simulink model "audio_project"  (R2022b)
settings: Solver=FixedStepDiscrete  StartTime=0.0  StopTime=inf  RelTol=1e-3
model workspace (MAT data in the model file):
  L = 5
  R = 0.5
  p = 2
libraries: audiosources x2, dspsnks4 x1
settings Model: Creator=The MathWorks, Inc.  LastModifiedBy=aymer
settings SolverCC: AlgebraicLoopSolver=TrustRegion  AutoInsertRateTranBlk=on
settings DataIOCC: LimitDataPoints=on  SaveOutput=off  SignalLogging=off  SaveTime=off  ReturnWorkspaceOutputs=off
settings OptimizationCC: LifeSpan=inf
settings DebuggingCC: AlgebraicLoopMsg=error  SingleTaskRateTransMsg=error  UnconnectedInputMsg=warning  UnconnectedOutputMsg=warning  UnconnectedLineMsg=warning  AllowSymbolicDim=off  SFUnexpectedBacktrackingDiag=warning  SFNoUnconditionalDefaultTransitionDiag=warning  SFExecutionAtInitializationDiag=none  SFMachineParentedDataDiag=warning  ArithmeticOperatorsInVariantConditions=warning
settings ModelReferenceCC: EnableRefExpFcnMdlSchedulingChecks=on
settings SFSimCC: SimUseLocalCustomCode=off  CustomCodeUndefinedFunction=UseInterfaceOnly
settings RTWCC: RTWUseLocalCustomCode=off
settings CodeAppCC: StateflowObjectComments=on
settings GRTTargetCC: TargetLangStandard=C89/C90 (ANSI)
settings ConfigComp: CovMetricSettings=dw  CovSaveCumulativeToWorkspaceVar=on  CovSaveSingleToWorkspaceVar=on  CovExternalEMLEnable=off  CovSFcnEnable=off

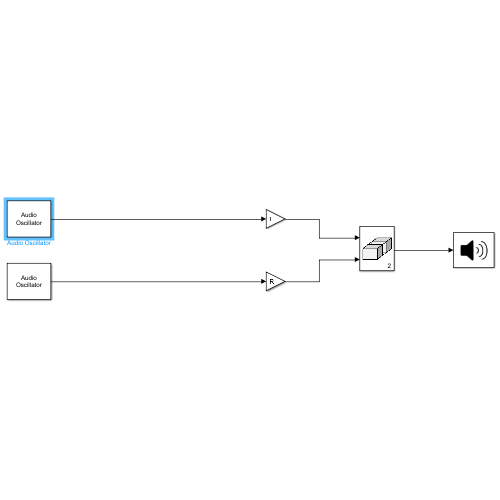
[thumbnail: Simulink's stored preview of the top-level diagram]
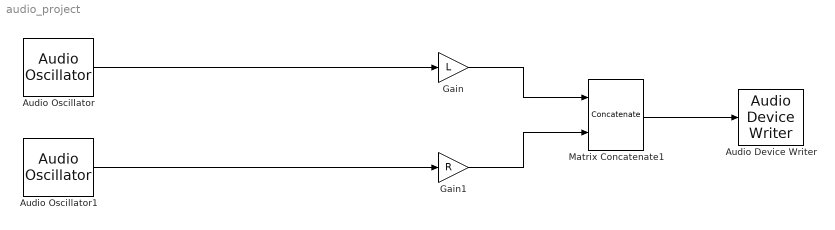
== system audio_project ==
  Audio Device Writer : dspsnks4/Audio Device Writer  Driver=DirectSound  Device=Speakers (Realtek High Definition Audio(SST))  InheritSampleRate=off  SampleRate=44100  BitDepth=16-bit integer  BufferSize=4096  NumBuffers=10  DefaultOutputChannelMapping=on  OutputChannelMapping=1:2  OutputNumUnderrunSamples=off  DriverIdx=1  DeviceWarnFlag=''
  Audio Oscillator : audiosources/Audio Oscillator  FrequencyPort=off  Frequency=1500  AmplitudePort=off  Amplitude=0  DCOffsetPort=off  PhaseOffset=0  DCOffset=0  WidthPort=off  Width=1  DutyCyclePort=off  DutyCycle=0.5  SampsPerFrame=512  Fs=44100  OutputDataType=double  SimulateUsing=Code generation
      settings: SignalType=sine
  Audio Oscillator1 : audiosources/Audio Oscillator  FrequencyPort=off  Frequency=1500  AmplitudePort=off  Amplitude=1  DCOffsetPort=off  PhaseOffset=0  DCOffset=0  WidthPort=off  Width=1  DutyCyclePort=off  DutyCycle=0.5  SampsPerFrame=512  Fs=44100  OutputDataType=double  SimulateUsing=Code generation
      settings: SignalType=sine
  Gain : Gain  Gain=L
  Gain1 : Gain  Gain=R
  Matrix Concatenate1 : Concatenate  Mode=Multidimensional array  ConcatenateDimension=2
  wires:
  Gain1/1 -> Matrix Concatenate1/2
  Gain/1 -> Matrix Concatenate1/1
  Matrix Concatenate1/1 -> Audio Device Writer/1
  Audio Oscillator1/1 -> Gain1/1
  Audio Oscillator/1 -> Gain/1
